simulink model "TwoRacercars_Kalman"  (R2022b)
settings: Solver=VariableStepAuto  StartTime=0.0  StopTime=10.0  RelTol=1e-3
values from neighbouring files (symbols this model uses):
  A = [0 1 0 0; 0 0 0 0; 0 0 0 1; 0 0 0 0]    [Racecar_Init.m]    (also in TwoRacecars_init.m = [0 1; 0 0])
  B = [0 0; 1 0; 0 0; 0 1]    [Racecar_Init.m]    (also in TwoRacecars_init.m = [0; 1])
  C = eye(2)    [TwoRacecars_init.m]
  K1 = lqr(A,B,Q1,R1)    [TwoRacecars_init.m]
  x0 = 0    [TwoRacecars_init.m]
  xd0 = 0    [TwoRacecars_init.m]
undefined symbols (not defined in the file or in its folder): Continuous, Time
libraries: simulink x4, ctrlSharedLib x2
settings Model: Creator=logan  LastModifiedBy=logan

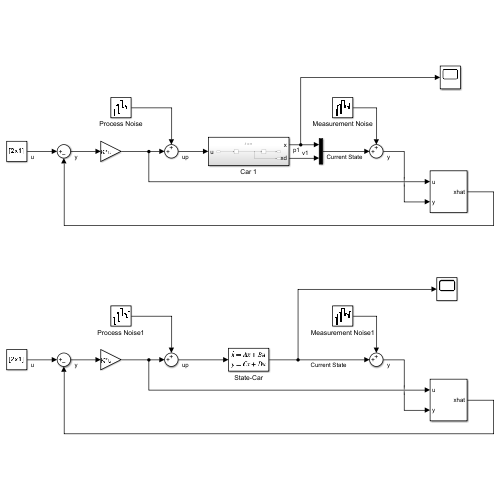
[thumbnail: Simulink's stored preview of the top-level diagram]
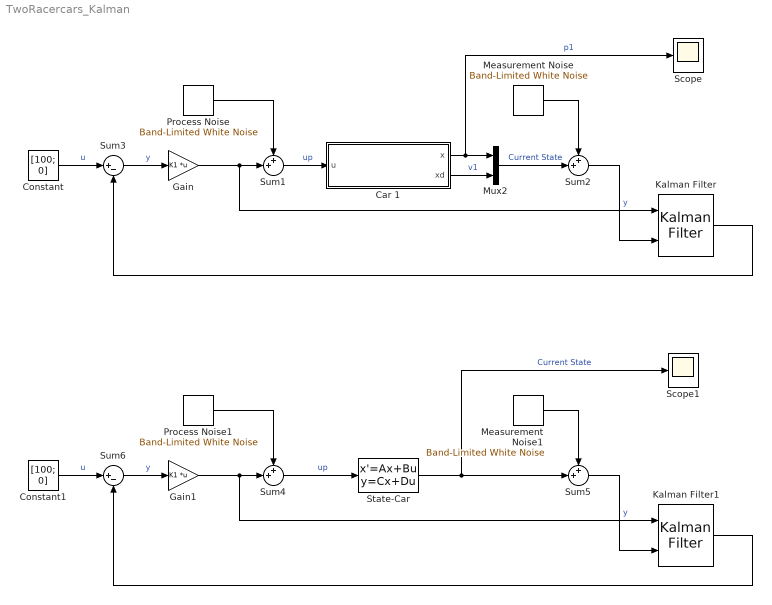
== system TwoRacercars_Kalman ==
  Car 1 : Subsystem
  Constant : Constant  Value=[100; 0]
  Constant1 : Constant  Value=[100; 0]
  Gain : Gain  Gain=K1  Multiplication=Matrix(K*u)
  Gain1 : Gain  Gain=K1  Multiplication=Matrix(K*u)
  Kalman Filter : ctrlSharedLib/Kalman Filter  TimeDomain=Continuous-Time  UseCurrentEstimator=on  ModelSource=Individual A, B, C, D matrices  ModelSourceVariable=Plant  A=A  B=B  C=C  D=0  NumberOfStates=1  NumberOfInputs=1  NumberOfOutputs=1  InitialEstimateSource=Dialog  X0=0  P0=10  UseK=off  UseGH=off  NumberOfProcessNoiseInputs=1  G=1  TimeInvariantG=on  H=0  TimeInvariantH=on  Q=0.1  TimeInvariantQ=on  R=0.1  TimeInvariantR=on  N=0  TimeInvariantN=on  AddInputPort=on  AddEnablePort=off  OutputEstimatedY=off  OutputP=off  Ts=-1
  Kalman Filter1 : ctrlSharedLib/Kalman Filter  TimeDomain=Continuous-Time  UseCurrentEstimator=on  ModelSource=Individual A, B, C, D matrices  ModelSourceVariable=Plant  A=A  B=B  C=C  D=0  NumberOfStates=1  NumberOfInputs=1  NumberOfOutputs=1  InitialEstimateSource=Dialog  X0=0  P0=10  UseK=off  UseGH=off  NumberOfProcessNoiseInputs=1  G=1  TimeInvariantG=on  H=0  TimeInvariantH=on  Q=0.1  TimeInvariantQ=on  R=0.1  TimeInvariantR=on  N=0  TimeInvariantN=on  AddInputPort=on  AddEnablePort=off  OutputEstimatedY=off  OutputP=off  Ts=-1
  Measurement Noise : simulink/Sources/Band-Limited White Noise  Cov=[0.1 0.1]  Ts=0.1  seed=[23341]
  Measurement Noise1 : simulink/Sources/Band-Limited White Noise  Cov=[0.1 0.1]  Ts=0.1  seed=[23341]
  Mux2 : Mux  Inputs=2
  Process Noise : simulink/Sources/Band-Limited White Noise  Cov=[0.1]  Ts=0.1  seed=[23341]
  Process Noise1 : simulink/Sources/Band-Limited White Noise  Cov=[0.1]  Ts=0.1  seed=[23341]
  Scope : Scope
  Scope1 : Scope
  State-Car : StateSpace  A=A  B=B  C=C  D=[0;0]  InitialCondition=0
  Sum{1..2,4..5} (4 alike) : Sum  Inputs=++|
  Sum3 : Sum  Inputs=|+-
  Sum6 : Sum  Inputs=|+-
  wires:
  Car 1/2(xd) -> Mux2/2  "v1"
  Car 1/1(x) -> Scope/1, Mux2/1  "p1"
  Mux2/1 -> Sum2/2  "Current State"
  Measurement Noise/1 -> Sum2/1
  Sum2/1 -> Kalman Filter/2  "y"
  Sum1/1 -> Car 1/1(u)  "up"
  Process Noise/1 -> Sum1/1
  Kalman Filter/1 -> Sum3/2
  Gain/1 -> Kalman Filter/1, Sum1/2
  Constant/1 -> Sum3/1  "u"
  Sum3/1 -> Gain/1  "y"
  Kalman Filter1/1 -> Sum6/2
  Constant1/1 -> Sum6/1  "u"
  Sum6/1 -> Gain1/1  "y"
  Gain1/1 -> Kalman Filter1/1, Sum4/2
  Process Noise1/1 -> Sum4/1
  Sum4/1 -> State-Car/1  "up"
  State-Car/1 -> Scope1/1, Sum5/2  "Current State"
  Sum5/1 -> Kalman Filter1/2  "y"
  Measurement Noise1/1 -> Sum5/1

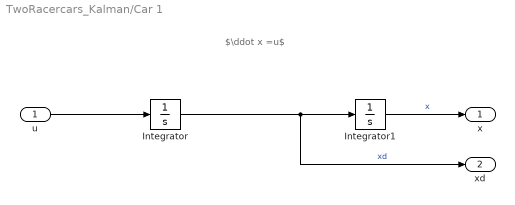
== system TwoRacercars_Kalman/Car 1 ==
  note: $\ddot x =u$
  u : Inport
  Integrator : Integrator  InitialCondition=xd0
  Integrator1 : Integrator  InitialCondition=x0
  x : Outport
  xd : Outport  Port=2
  wires:
  Integrator/1 -> xd/1, Integrator1/1  "xd"
  Integrator1/1 -> x/1  "x"
  u/1 -> Integrator/1
